simulink model "Q5"  (R2020b)
settings: Solver=VariableStepAuto  StartTime=0.0  StopTime=30  RelTol=1e-3
undefined symbols (not defined in the file): A_num, B_num, C_num, K_fast, K_slow, L_obs
settings Model: Creator=asus  LastModifiedBy=asus

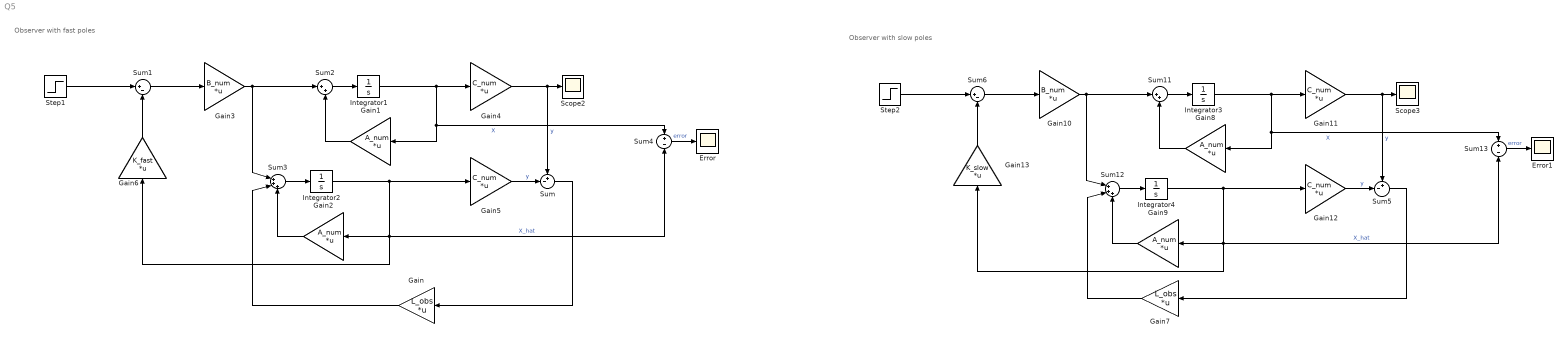
== system Q5 ==
  note: Observer with fast poles
  note: Observer with slow poles
  Error : Scope
  Error1 : Scope
  Gain : Gain  Gain=L_obs  Multiplication=Matrix(K*u)
  Gain{1..2,8..9} (4 alike) : Gain  Gain=A_num  Multiplication=Matrix(K*u)
  Gain10 : Gain  Gain=B_num  Multiplication=Matrix(K*u)
  Gain{4..5,11..12} (4 alike) : Gain  Gain=C_num  Multiplication=Matrix(K*u)
  Gain13 : Gain  Gain=K_slow  Multiplication=Matrix(K*u)
  Gain3 : Gain  Gain=B_num  Multiplication=Matrix(K*u)
  Gain6 : Gain  Gain=K_fast  Multiplication=Matrix(K*u)
  Gain7 : Gain  Gain=L_obs  Multiplication=Matrix(K*u)
  Integrator{1..4} (4 alike) : Integrator
  Scope2 : Scope
  Scope3 : Scope
  Step1 : Step  SampleTime=0
  Step2 : Step  SampleTime=0
  Sum : Sum  Inputs=+-|
  Sum1 : Sum  Inputs=|+-
  Sum11 : Sum  Inputs=|++
  Sum12 : Sum  Inputs=|+++
  Sum13 : Sum  Inputs=+|-
  Sum2 : Sum  Inputs=|++
  Sum3 : Sum  Inputs=|+++
  Sum4 : Sum  Inputs=+|-
  Sum5 : Sum  Inputs=+-|
  Sum6 : Sum  Inputs=|+-
  wires:
  Gain7/1 -> Sum12/2
  Gain3/1 -> Sum3/1, Sum2/1
  Integrator2/1 -> Gain5/1, Sum4/2, Gain6/1, Gain2/1  "X_hat"
  Step2/1 -> Sum6/1
  Gain5/1 -> Sum/2  "y"
  Gain/1 -> Sum3/2
  Sum3/1 -> Integrator2/1
  Gain10/1 -> Sum12/1, Sum11/1
  Gain6/1 -> Sum1/2
  Sum11/1 -> Integrator3/1
  Sum6/1 -> Gain10/1
  Gain12/1 -> Sum5/2  "y"
  Gain2/1 -> Sum3/3
  Gain8/1 -> Sum11/2
  Gain13/1 -> Sum6/2
  Sum5/1 -> Gain7/1
  Gain9/1 -> Sum12/3
  Step1/1 -> Sum1/1
  Integrator3/1 -> Gain11/1, Sum13/1, Gain8/1  "X"
  Gain11/1 -> Sum5/1, Scope3/1  "y"
  Integrator1/1 -> Gain4/1, Sum4/1, Gain1/1  "X"
  Sum12/1 -> Integrator4/1
  Gain4/1 -> Sum/1, Scope2/1  "y"
  Sum4/1 -> Error/1  "error"
  Sum13/1 -> Error1/1  "error"
  Gain1/1 -> Sum2/2
  Integrator4/1 -> Gain12/1, Sum13/2, Gain13/1, Gain9/1  "X_hat"
  Sum1/1 -> Gain3/1
  Sum2/1 -> Integrator1/1
  Sum/1 -> Gain/1
